simulink model "joystick_test"  (Simulink 8.0)
settings: Solver=ode45  StartTime=0.0  StopTime=10.0  RelTol=1e-3
libraries: aerolibanimutils x1
settings Model: Creator=mufasa  LastModifiedBy=mufasa

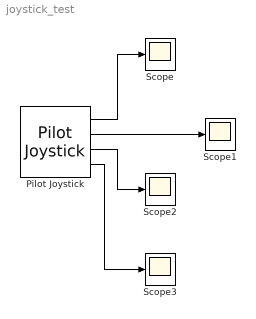
== system joystick_test ==
  Pilot Joystick : aerolibanimutils/Pilot Joystick  JoystickID=Joystick1  OutputConfiguration=FourAxis  SampleTime=1/30
  Scope{,1..3} (4 alike) : Scope
      Scope2 settings: SaveName=ScopeData2
      Scope3 settings: SaveName=ScopeData3
  wires:
  Pilot Joystick/1 -> Scope/1
  Pilot Joystick/2 -> Scope1/1
  Pilot Joystick/3 -> Scope2/1
  Pilot Joystick/4 -> Scope3/1
